simulink library "fuselage_ul"  (R2018b)
settings: Solver=VariableStepAuto  StartTime=0.0  StopTime=10.0  RelTol=1e-3
settings Model: Creator=mcobb  LastModifiedBy=mcobb

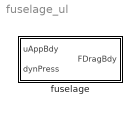
== system fuselage_ul ==
  fuselage : Subsystem  mask{len=0, diam=0, sideCD=0, endCD=0}
      mask prompts: len "Length"; diam "Diameter"; sideCD "Sideways drag coeff"; endCD "End-ways drag coeff"

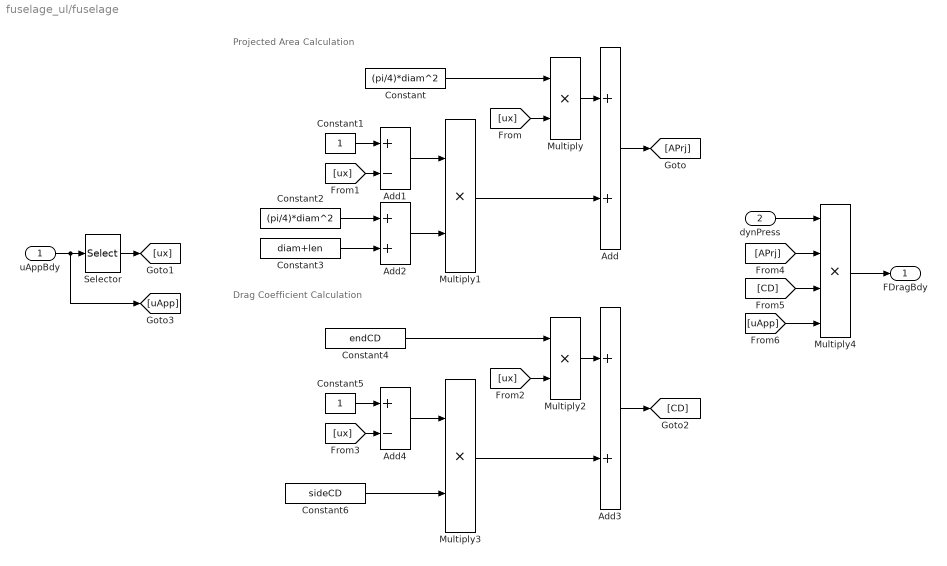
== system fuselage_ul/fuselage ==
  note: Drag Coefficient Calculation
  note: Projected Area Calculation
  uAppBdy : Inport
  dynPress : Inport  Port=2
  Add : Sum
  Add1 : Sum  Inputs=+-
  Add2 : Sum
  Add3 : Sum
  Add4 : Sum  Inputs=+-
  Constant : Constant  Value=(pi/4)*diam^2
  Constant1 : Constant
  Constant2 : Constant  Value=(pi/4)*diam^2
  Constant3 : Constant  Value=diam+len
  Constant4 : Constant  Value=endCD
  Constant5 : Constant
  Constant6 : Constant  Value=sideCD
  Multiply{,1..3} (4 alike) : Product
  Multiply4 : Product  Inputs=4
  Selector : Selector  InputPortWidth=3  IndexOptions=Index vector (dialog)  Indices=1  OutputSizes=1
  FDragBdy : Outport
  wires:
  uAppBdy/1 -> [uApp], Selector/1
  Add/1 -> [APrj]
  Selector/1 -> [ux]
  Multiply1/1 -> Add/2
  Multiply/1 -> Add/1
  Constant/1 -> Multiply/1
  [ux] -> Multiply/2
  Add1/1 -> Multiply1/1
  Constant1/1 -> Add1/1
  [ux] -> Add1/2
  Add2/1 -> Multiply1/2
  Constant2/1 -> Add2/1
  Constant3/1 -> Add2/2
  [ux] -> Add4/2
  Constant5/1 -> Add4/1
  Add4/1 -> Multiply3/1
  [ux] -> Multiply2/2
  Multiply2/1 -> Add3/1
  Multiply3/1 -> Add3/2
  Constant6/1 -> Multiply3/2
  Constant4/1 -> Multiply2/1
  Add3/1 -> [CD]
  Multiply4/1 -> FDragBdy/1
  dynPress/1 -> Multiply4/1
  [APrj] -> Multiply4/2
  [CD] -> Multiply4/3
  [uApp] -> Multiply4/4
